simulink subsystem "subref_compute_desaturation_gain"  (R2024b)
settings: Solver=VariableStepAuto  StartTime=0.0  StopTime=10.0  RelTol=1e-3
libraries: simulink x4
settings Model: Creator=CETCA  LastModifiedBy=CETCA

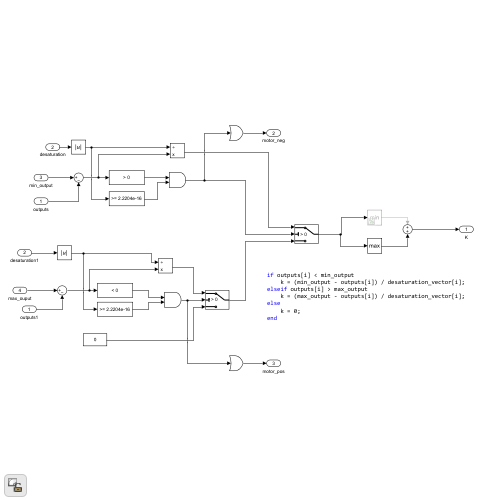
[thumbnail: Simulink's stored preview of the top-level diagram]
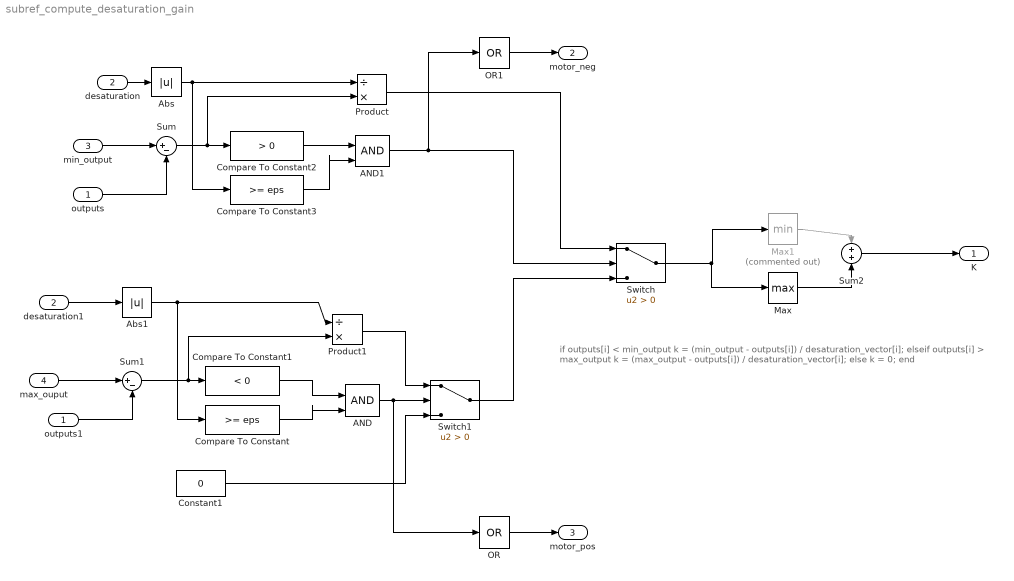
== system subref_compute_desaturation_gain ==
  note: if outputs[i] < min_output
      | k = (min_output - outputs[i]) / desaturation_vector[i];
      | elseif outputs[i] > max_output
      | k = (max_output - outputs[i]) / desaturation_vector[i];
      | else
      | k = 0;
      | end
  outputs : Inport
  desaturation : Inport  Port=2
  min_output : Inport  Port=3
  max_ouput : Inport  Port=4
  AND : Logic  IconShape=distinctive  AllPortsSameDT=off  OutDataTypeStr=boolean
  AND1 : Logic  IconShape=distinctive  AllPortsSameDT=off  OutDataTypeStr=boolean
  Abs : Abs  SaturateOnIntegerOverflow=off
  Abs1 : Abs  SaturateOnIntegerOverflow=off
  Compare To Constant : simulink/Logic and Bit Operations/Compare To Constant  relop=>=  const=eps  OutDataTypeStr=boolean
  Compare To Constant1 : simulink/Logic and Bit Operations/Compare To Constant  relop=<  const=0  OutDataTypeStr=boolean
  Compare To Constant2 : simulink/Logic and Bit Operations/Compare To Constant  relop=>  const=0  OutDataTypeStr=boolean
  Compare To Constant3 : simulink/Logic and Bit Operations/Compare To Constant  relop=>=  const=eps  OutDataTypeStr=boolean
  Constant1 : Constant  Value=0
  Max : MinMax  Function=max
  Max1 : MinMax  Commented=on
  OR : Logic  Operator=OR  Inputs=1  IconShape=distinctive  AllPortsSameDT=off  OutDataTypeStr=boolean
  OR1 : Logic  Operator=OR  Inputs=1  IconShape=distinctive  AllPortsSameDT=off  OutDataTypeStr=boolean
  Product : Product  Inputs=/*
  Product1 : Product  Inputs=/*
  Sum : Sum  Inputs=|+-
  Sum1 : Sum  Inputs=|+-
  Sum2 : Sum  Inputs=2
  Switch : Switch  Criteria=u2 > Threshold  SaturateOnIntegerOverflow=off  InputSameDT=off
  Switch1 : Switch  Criteria=u2 > Threshold  SaturateOnIntegerOverflow=off  InputSameDT=off
  desaturation1 : InportShadow  Port=2
  outputs1 : InportShadow
  K : Outport
  motor_neg : Outport  Port=2
  motor_pos : Outport  Port=3
  wires:
  desaturation/1 -> Abs/1
  outputs/1 -> Sum/2
  min_output/1 -> Sum/1
  Sum/1 -> Compare To Constant2/1, Product/2
  Abs/1 -> Compare To Constant3/1, Product/1
  Product/1 -> Switch/1
  desaturation1/1 -> Abs1/1
  Abs1/1 -> Product1/1, Compare To Constant/1
  Switch1/1 -> Switch/3
  AND/1 -> Switch1/2, OR/1
  Compare To Constant/1 -> AND/2
  Sum1/1 -> Compare To Constant1/1, Product1/2
  Compare To Constant1/1 -> AND/1
  Compare To Constant2/1 -> AND1/1
  AND1/1 -> Switch/2, OR1/1
  Compare To Constant3/1 -> AND1/2
  Constant1/1 -> Switch1/3
  Product1/1 -> Switch1/1
  max_ouput/1 -> Sum1/1
  outputs1/1 -> Sum1/2
  OR/1 -> motor_pos/1
  OR1/1 -> motor_neg/1
  Sum2/1 -> K/1
  Switch/1 -> Max1/1, Max/1
  Max1/1 -> Sum2/1
  Max/1 -> Sum2/2
